simulink model "oneshotadder"  (R2022b)
settings: Solver=FixedStepAuto  StartTime=0.0  StopTime=inf  FixedStep=0.5  RelTol=1e-3
undefined symbols (not defined in the file): m, n, sigbuilder_block
libraries: robotlib x7
settings Model: Creator=ivory  LastModifiedBy=sprinkle
settings SolverCC: AlgebraicLoopSolver=TrustRegion
settings OptimizationCC: EnhancedBackFolding=on  PassReuseOutputArgsThreshold=0  MaxStackSize=64  OptimizeBlockOrder=speed  DifferentSizesBufferReuse=on  OptimizationCustomize=off
settings DebuggingCC: ParameterTunabilityLossMsg=error  UnconnectedInputMsg=warning  UnconnectedOutputMsg=warning  UnconnectedLineMsg=warning  SFMachineParentedDataDiag=warning
settings HardwareCC: ProdBitPerPointer=32  ProdBitPerSizeT=32  ProdBitPerPtrDiffT=32  ProdLargestAtomicFloat=None  ProdIntDivRoundTo=Undefined  ProdEndianess=Unspecified  ProdWordSize=32  ProdHWDeviceType=Generic->Unspecified (assume 32-bit Generic)  UseEmbeddedCoderFeatures=off
settings ModelReferenceCC: EnableRefExpFcnMdlSchedulingChecks=on
settings SFSimCC: MATLABDynamicMemAlloc=off  SimTargetLang=C++
settings RTWCC: Description=Embedded Coder  SystemTargetFile=ert.tlc  HardwareBoard=Robot Operating System (ROS)  TLCOptions="-aInlineSetEventsForThisBaseRateFcn=TLC_FALSE -aSuppressMultiTaskScheduler=TLC_FALSE  -aRateBasedStepFcn=0"  TemplateMakefile=ert_default_tmf  Toolchain=Catkin  TargetLang=C++
settings CodeAppCC: ForceParamTrailComments=on  OperatorAnnotations=on
settings ERTTargetCC: ERTCustomFileBanners=off  SupportContinuousTime=on  SupportNonInlinedSFcns=on  RemoveResetFunc=off  ModelStepFunctionPrototypeControlCompliant=off

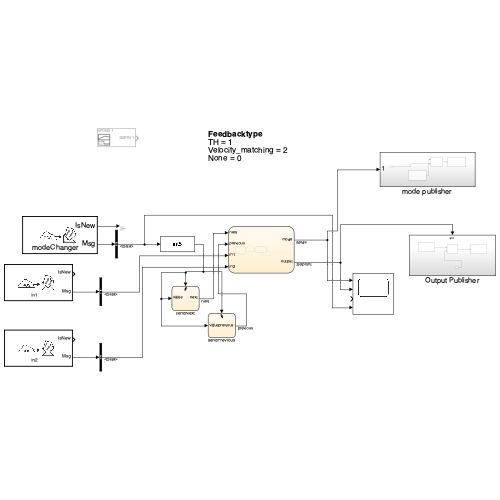
[thumbnail: Simulink's stored preview of the top-level diagram]
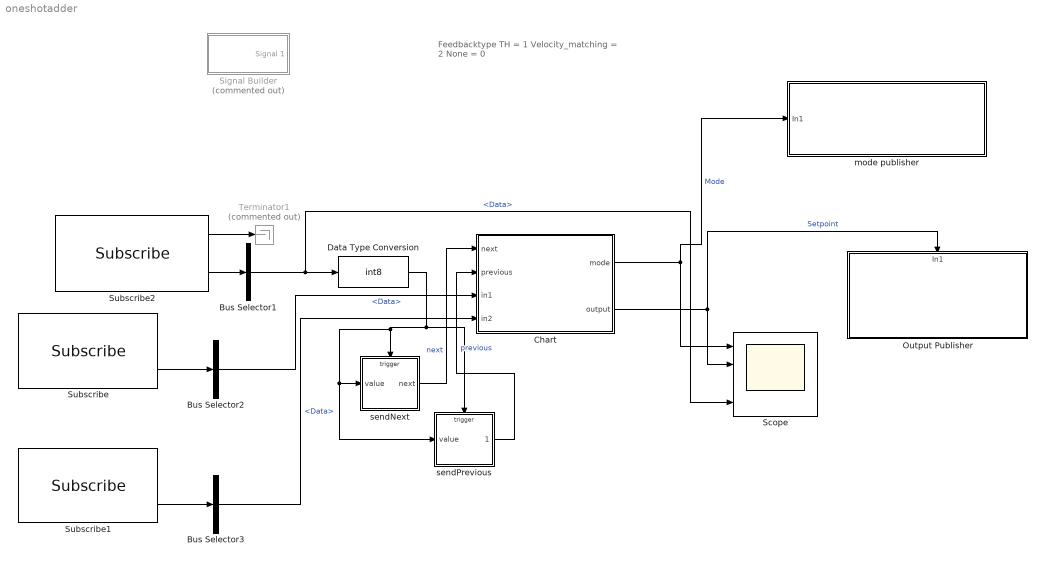
== system oneshotadder ==
  note: Feedbacktype
      | TH = 1
      | Velocity_matching = 2
      | None = 0
  Bus Selector1 : BusSelector  DialogController=Simulink.DDGSource_BusSelector  OutputSignals=Data
  Bus Selector2 : BusSelector  DialogController=Simulink.DDGSource_BusSelector  OutputSignals=Data
  Bus Selector3 : BusSelector  DialogController=Simulink.DDGSource_BusSelector  OutputSignals=Data
  Chart : Stateflow chart  TreatAsAtomicUnit=on
  Data Type Conversion : DataTypeConversion  OutDataTypeStr=int8  SaturateOnIntegerOverflow=off  RndMeth=Floor
  Output Publisher : Subsystem
      settings: PortSchema="{\"entries\":[{\"content\":{\"sides\":[{\"content\":{\"connectorIds\":[]},\"type\":\"ConnectorPlacement.EquallySpacedRectSide\",\"uuid\":\"7228cb39-d042-4544-9404-c470f4fdfbf1\"},{\"content\":{\"connectorIds\":[],\"side\":\"RIGHT\"},\"type\":\"ConnectorPlacement.EquallySpacedRectSide\",\"uuid\":\"d3b4c5d4-5a27-4f35-aed9-956300822ff3\"},{\"content\":{\"connectorIds\":[\"In1\"],\"side\":\"TOP\"},\"type\":\"ConnectorPlacement.EquallySpacedRectSide\",\"uuid\":\"960bf3c5-2ad7-4c01-a07e-903e5f41e994\"},{\"content\":{\"connectorIds\":[],\"side\":\"BOTTOM\"},\"type\":\"ConnectorPlacement.EquallySpacedRectSide\",\"uuid\":\"1493639f-9397-4233-abc9-2a06b786f373\"}]},\"type\":\"ConnectorPlacement.EquallySpacedConnector\",\"uuid\":\"6b7d05b9-818d-4613-8d2a-25b4b7d7d80b\"}],\"packageUris\":[\"http://schema.mathworks.com/mf0/Connector/19700101\"],\"version\":\"1.0\"}"
  Scope : Scope  NumInputPorts=4
  Signal Builder : Subsystem  Tag=STV Subsys  Commented=on  LoadFcn=sigbuilder_block('load');  StartFcn=sigbuilder_block('start');  StopFcn=sigbuilder_block('stop');  ClipboardFcn=sigbuilder_block('clipboard');  mask(Sigbuilder block){tuvar=[0:10]}
      mask help: Simulink:masks:SigbuilderBlock_MD
      mask init:
      | if ~strcmp(get_param(bdroot(gcbh),'SimulationStatus'),'stopped') tuvar = sigbuilder_block('maskInit'); end
      settings: CopyFcn=sigbuilder_block('copy');  DeleteFcn=sigbuilder_block('delete');  ModelCloseFcn=sigbuilder_block('modelClose');  PreSaveFcn=sigbuilder_block('preSave');  PauseFcn=sigbuilder_block('pause');  ContinueFcn=sigbuilder_block('continue');  NameChangeFcn=sigbuilder_block('namechange');  OpenFcn=sigbuilder_block('open',[0 35.25 1440 692.25 ]);  CloseFcn=sigbuilder_block('close');
      mask Display: plot(0, 0, 100, 100,[2, 2, 32, 32, 2], [68, 8, 8, 68, 68],[32, 2], [38, 38], [32, 19, 2],[53, 60, 44], [32, 17, 17, 2],[16, 16, 31, 31]);txt = getActiveGroup(gcbh);text(2, 100, txt,'verticalAlignment', 'top');
  Subscribe : robotlib/Subscribe  topicSource=Specify your own  topic=in1  messageType=std_msgs/Float64  SampleTime=-1  legacyBusStruct=off  messageQueueLength=1
      settings: LibrarySourceBlock=roslib/ROS/Subscribe
  Subscribe1 : robotlib/Subscribe  topicSource=Specify your own  topic=in2  messageType=std_msgs/Float64  SampleTime=-1  legacyBusStruct=off  messageQueueLength=1
      settings: LibrarySourceBlock=roslib/ROS/Subscribe
  Subscribe2 : robotlib/Subscribe  topicSource=Specify your own  topic=modeChanger  messageType=std_msgs/Int8  SampleTime=-1  legacyBusStruct=off  messageQueueLength=1
  Terminator1 : Terminator  Commented=on
  mode publisher : Subsystem
  sendNext : Stateflow chart  TreatAsAtomicUnit=on
  sendPrevious : Stateflow chart  TreatAsAtomicUnit=on
  wires:
  Subscribe2/1 -> Terminator1/1
  Subscribe2/2 -> Bus Selector1/1
  Chart/1(mode) -> mode publisher/1(In1), Scope/1  "Mode"
  Chart/2(output) -> Output Publisher/1(In1), Scope/2  "Setpoint"
  sendNext/1(next) -> Chart/1(next)  "next"
  sendPrevious/1(previous) -> Chart/2(previous)  "previous"
  Data Type Conversion/1 -> sendPrevious/Trigger, sendPrevious/1(value), sendNext/1(value), sendNext/Trigger
  Bus Selector1/1 -> Scope/4, Data Type Conversion/1  "<Data>"
  Subscribe/2 -> Bus Selector2/1
  Subscribe1/2 -> Bus Selector3/1
  Bus Selector2/1 -> Chart/3(in1)  "<Data>"
  Bus Selector3/1 -> Chart/4(in2)  "<Data>"

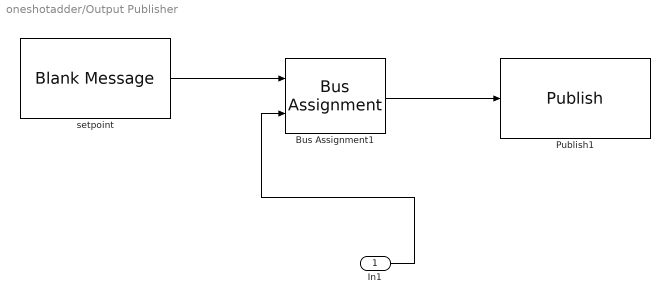
== system oneshotadder/Output Publisher ==
  In1 : Inport
  Bus Assignment1 : BusAssignment  AssignedSignals=Data
  Publish1 : robotlib/Publish  topicSource=Specify your own  topic=output  messageType=std_msgs/Float64  legacyBusStruct=off  messageQueueLength=1
  setpoint : robotlib/Blank Message  messageClass=Message  entityType=std_msgs/Float64  messageType=std_msgs/Float64  SampleTime=-1  legacyBusStruct=off
  wires:
  Bus Assignment1/1 -> Publish1/1
  setpoint/1 -> Bus Assignment1/1
  In1/1 -> Bus Assignment1/2

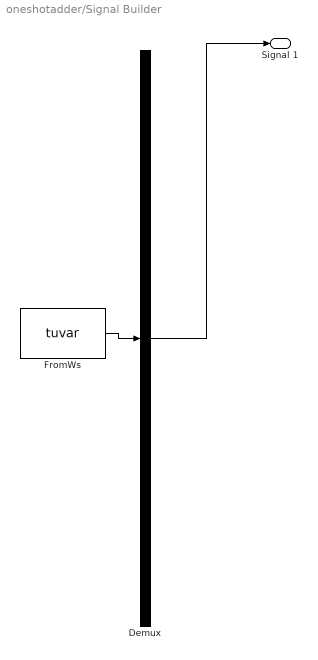
== system oneshotadder/Signal Builder ==
  Demux : Demux  Tag=STV Demux  Outputs=1
      settings: DisplayOption=none
  FromWs : FromWorkspace  Tag=STV FromWs  VariableName=tuvar
      SigBuilderData=|
      | common.afterFinalStr = 'Extrapolate'
      | common.sampleTime = 0
      | dataSet.timeRange = [0 1800]
      | dataSet.name = 'Group 1'
      | sbobj.Groups.Name = 'Group 1'
      | sbobj.Groups.Signals.Name = 'Signal 1'
      | sbobj.Groups.Signals.XData = [0 0.0134060382843 0.0270323753357 0.0364005565643 0.0445430278778 0.0529842376709 0.0616769790649 0.0696005821228 0.0774240493774 0.086790561676 0.0956425666809 0.104114532471 ... (122718 elements, 1x122718)]
      | sbobj.Groups.Signals.YData = [0 0 0 0 0 0 0 0 0 0 0 0 ... (122718 elements, 1x122718)]
      | sbobj.Groups.TimeRange = [0 1800]
  Signal 1 : Outport  Tag=STV Outport
  wires:
  FromWs/1 -> Demux/1
  Demux/1 -> Signal 1/1

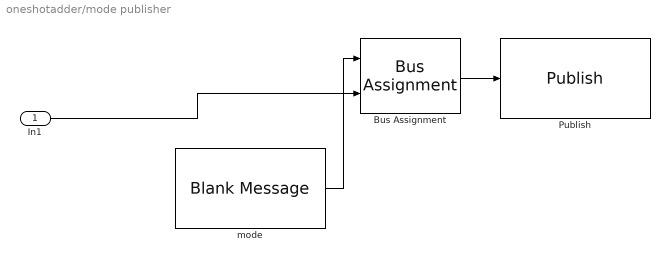
== system oneshotadder/mode publisher ==
  In1 : Inport
  Bus Assignment : BusAssignment  AssignedSignals=Data
  Publish : robotlib/Publish  topicSource=Specify your own  topic=mode  messageType=std_msgs/UInt8  legacyBusStruct=off  messageQueueLength=1
  mode : robotlib/Blank Message  messageClass=Message  entityType=std_msgs/UInt8  messageType=std_msgs/UInt8  SampleTime=-1  legacyBusStruct=off
  wires:
  Bus Assignment/1 -> Publish/1
  mode/1 -> Bus Assignment/1
  In1/1 -> Bus Assignment/2

== stateflow chart oneshotadder/Chart ==
  note: Mode 1 = Waiting for input
      | Mode 2 = Triggered
  state Init
    entry: mode =1;
    output  = -1;
  state Const_th
    entry: mode = 2;
  Init -> Const_th : next{output=in1+in2}
  (default) -> Init
  Const_th -> Const_th [order 1] : next{output=in1+in2}
  Const_th -> Init [order 2] : previous
  data: mode output uint8; output output double; next input; previous input; in1 input; in2 input

== stateflow chart oneshotadder/sendNext ==
  state idle
    during:
    if checkHigh(value)
    next.data = 1;
    send(next)
    end
  (default) -> idle
  data: data function_input; result function_output; next output; value input int8
  events: event input RISING_EDGE_EVENT
  function result = checkHigh(data):
    | function result = checkHigh(data)
    | 
    | if data == 1
    |     result = 1;
    | else
    |     result = 0;
    | end
    | 
    | end

== stateflow chart oneshotadder/sendPrevious ==
  state idle
    during:
    if checkLow(value)
    previous.data = 1;
    send(previous)
    end
  (default) -> idle
  data: data function_input; result function_output; previous output; value input int8
  events: event input FALLING_EDGE_EVENT
  function result = checkLow(data):
    | function result = checkLow(data)
    | 
    | if data == -1
    |     result = 1;
    | else
    |     result = 0;
    | end
    | 
    | end
